simulink model "Adder8bit"  (R2016a)
settings: Solver=VariableStepAuto  StartTime=0.0  StopTime=10.0  RelTol=1e-3
libraries: hdlsllib x17
settings Model: Creator=duyvu  LastModifiedBy=duyvu

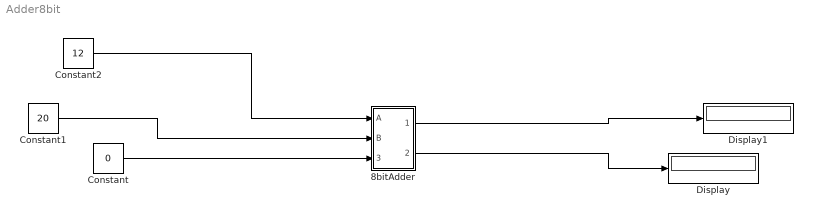
== system Adder8bit ==
  8bitAdder : Subsystem
  Constant : Constant  Value=0  OutDataTypeStr=boolean
  Constant1 : Constant  Value=20  OutDataTypeStr=int8
  Constant2 : Constant  Value=12  OutDataTypeStr=int8
  Display : Display
  Display1 : Display
  wires:
  Constant2/1 -> 8bitAdder/1(A)
  Constant1/1 -> 8bitAdder/2(B)
  Constant/1 -> 8bitAdder/3(CIn)
  8bitAdder/1(Carry) -> Display1/1
  8bitAdder/2(Sum) -> Display/1

== system Adder8bit/8bitAdder ==
  A : Inport  OutDataTypeStr=int8
  B : Inport  Port=2
  CIn : Inport  Port=3
  Bit Concat : hdlsllib/HDL Operations/Bit Concat  numInputs=8
  Data Type Conversion : DataTypeConversion  OutDataTypeStr=int8
  Subsystem10 : Subsystem
  Carry : Outport
  Sum : Outport  Port=2
  wires:
  Data Type Conversion/1 -> Sum/1
  Bit Concat/1 -> Data Type Conversion/1
  Subsystem10/2(Carry) -> Carry/1
  Subsystem10/5(Out3) -> Bit Concat/5
  Subsystem10/6(Out4) -> Bit Concat/4
  Subsystem10/7(Out5) -> Bit Concat/3
  Subsystem10/3(Out1) -> Bit Concat/7
  Subsystem10/4(Out2) -> Bit Concat/6
  B/1 -> Subsystem10/2(B)
  CIn/1 -> Subsystem10/3(CIn)
  A/1 -> Subsystem10/1(A)
  Subsystem10/1(Out0) -> Bit Concat/8
  Subsystem10/8(Out6) -> Bit Concat/2
  Subsystem10/9(Out7) -> Bit Concat/1

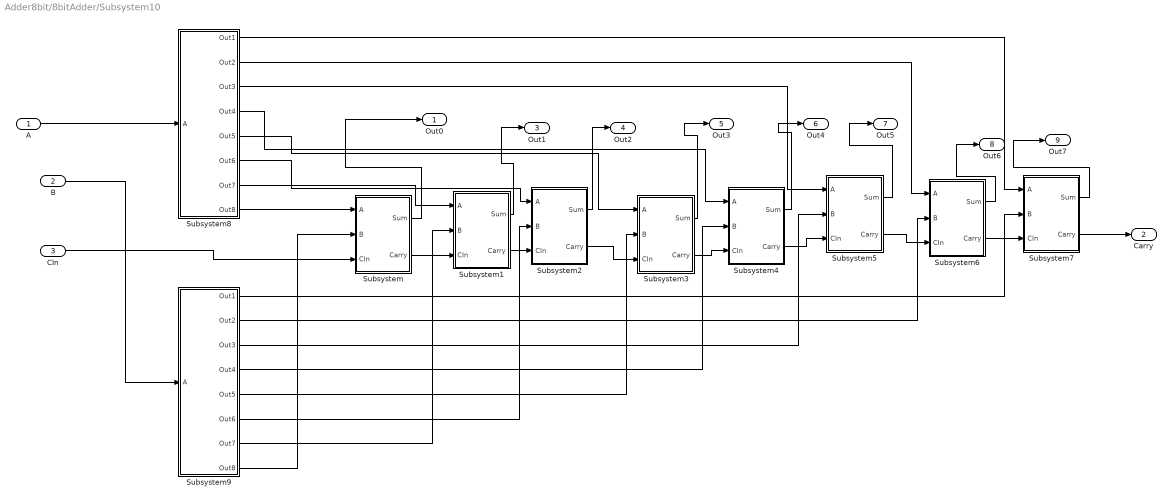
== system Adder8bit/8bitAdder/Subsystem10 ==
  A : Inport  OutDataTypeStr=int8
  B : Inport  Port=2
  CIn : Inport  Port=3
  Subsystem : Subsystem
  Subsystem1 : Subsystem
  Subsystem2 : Subsystem
  Subsystem3 : Subsystem
  Subsystem4 : Subsystem
  Subsystem5 : Subsystem
  Subsystem6 : Subsystem
  Subsystem7 : Subsystem
  Subsystem8 : Subsystem
  Subsystem9 : Subsystem
  Out0 : Outport  OutDataTypeStr=boolean
  Carry : Outport  Port=2
  Out1 : Outport  Port=3  OutDataTypeStr=boolean
  Out2 : Outport  Port=4  OutDataTypeStr=boolean
  Out3 : Outport  Port=5
  Out4 : Outport  Port=6
  Out5 : Outport  Port=7
  Out6 : Outport  Port=8
  Out7 : Outport  Port=9
  wires:
  B/1 -> Subsystem9/1(A)
  Subsystem8/3(Out3) -> Subsystem5/1(A)
  Subsystem8/2(Out2) -> Subsystem6/1(A)
  Subsystem8/7(Out7) -> Subsystem1/1(A)
  Subsystem8/5(Out5) -> Subsystem3/1(A)
  Subsystem8/8(Out8) -> Subsystem/1(A)
  Subsystem8/6(Out6) -> Subsystem2/1(A)
  Subsystem8/4(Out4) -> Subsystem4/1(A)
  Subsystem3/1(Sum) -> Out3/1
  A/1 -> Subsystem8/1(A)
  Subsystem6/1(Sum) -> Out6/1
  Subsystem9/5(Out5) -> Subsystem3/2(B)
  Subsystem5/1(Sum) -> Out5/1
  Subsystem4/1(Sum) -> Out4/1
  Subsystem8/1(Out1) -> Subsystem7/1(A)
  Subsystem7/1(Sum) -> Out7/1
  Subsystem9/8(Out8) -> Subsystem/2(B)
  Subsystem9/4(Out4) -> Subsystem4/2(B)
  Subsystem7/2(Carry) -> Carry/1
  Subsystem/2(Carry) -> Subsystem1/3(CIn)
  Subsystem1/1(Sum) -> Out1/1
  Subsystem2/2(Carry) -> Subsystem3/3(CIn)
  Subsystem1/2(Carry) -> Subsystem2/3(CIn)
  Subsystem/1(Sum) -> Out0/1
  CIn/1 -> Subsystem/3(CIn)
  Subsystem2/1(Sum) -> Out2/1
  Subsystem3/2(Carry) -> Subsystem4/3(CIn)
  Subsystem9/7(Out7) -> Subsystem1/2(B)
  Subsystem9/6(Out6) -> Subsystem2/2(B)
  Subsystem4/2(Carry) -> Subsystem5/3(CIn)
  Subsystem9/1(Out1) -> Subsystem7/2(B)
  Subsystem9/2(Out2) -> Subsystem6/2(B)
  Subsystem9/3(Out3) -> Subsystem5/2(B)
  Subsystem5/2(Carry) -> Subsystem6/3(CIn)
  Subsystem6/2(Carry) -> Subsystem7/3(CIn)

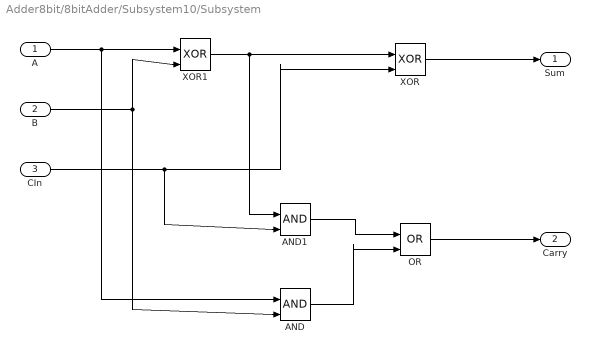
== system Adder8bit/8bitAdder/Subsystem10/Subsystem ==
  A : Inport
  B : Inport  Port=2
  CIn : Inport  Port=3
  AND : Logic  IconShape=distinctive  AllPortsSameDT=off  OutDataTypeStr=boolean
  AND1 : Logic  IconShape=distinctive  AllPortsSameDT=off  OutDataTypeStr=boolean
  "OR " : Logic  Operator=OR  IconShape=distinctive  AllPortsSameDT=off  OutDataTypeStr=boolean
  XOR : Logic  Operator=XOR  IconShape=distinctive  AllPortsSameDT=off  OutDataTypeStr=boolean
  XOR1 : Logic  Operator=XOR  IconShape=distinctive  AllPortsSameDT=off  OutDataTypeStr=boolean
  Sum : Outport
  Carry : Outport  Port=2
  wires:
  CIn/1 -> XOR/2, AND1/2
  XOR1/1 -> AND1/1, XOR/1
  A/1 -> XOR1/1, AND/1
  AND1/1 -> "OR "/1
  XOR/1 -> Sum/1
  B/1 -> AND/2, XOR1/2
  "OR "/1 -> Carry/1
  AND/1 -> "OR "/2

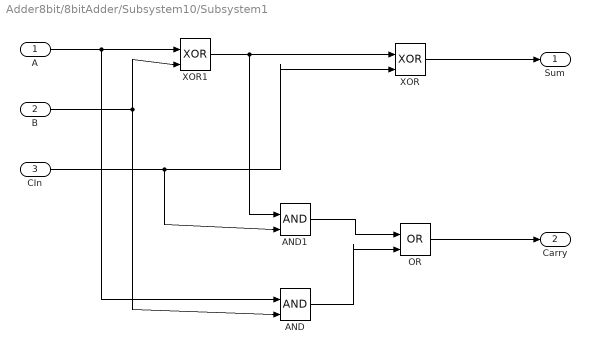
== system Adder8bit/8bitAdder/Subsystem10/Subsystem1 ==
  A : Inport
  B : Inport  Port=2
  CIn : Inport  Port=3
  AND : Logic  IconShape=distinctive  AllPortsSameDT=off  OutDataTypeStr=boolean
  AND1 : Logic  IconShape=distinctive  AllPortsSameDT=off  OutDataTypeStr=boolean
  "OR " : Logic  Operator=OR  IconShape=distinctive  AllPortsSameDT=off  OutDataTypeStr=boolean
  XOR : Logic  Operator=XOR  IconShape=distinctive  AllPortsSameDT=off  OutDataTypeStr=boolean
  XOR1 : Logic  Operator=XOR  IconShape=distinctive  AllPortsSameDT=off  OutDataTypeStr=boolean
  Sum : Outport
  Carry : Outport  Port=2
  wires:
  CIn/1 -> XOR/2, AND1/2
  XOR1/1 -> AND1/1, XOR/1
  A/1 -> XOR1/1, AND/1
  AND1/1 -> "OR "/1
  XOR/1 -> Sum/1
  B/1 -> AND/2, XOR1/2
  "OR "/1 -> Carry/1
  AND/1 -> "OR "/2

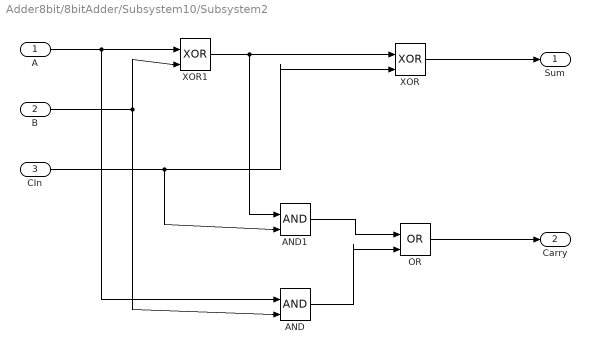
== system Adder8bit/8bitAdder/Subsystem10/Subsystem2 ==
  A : Inport
  B : Inport  Port=2
  CIn : Inport  Port=3
  AND : Logic  IconShape=distinctive  AllPortsSameDT=off  OutDataTypeStr=boolean
  AND1 : Logic  IconShape=distinctive  AllPortsSameDT=off  OutDataTypeStr=boolean
  "OR " : Logic  Operator=OR  IconShape=distinctive  AllPortsSameDT=off  OutDataTypeStr=boolean
  XOR : Logic  Operator=XOR  IconShape=distinctive  AllPortsSameDT=off  OutDataTypeStr=boolean
  XOR1 : Logic  Operator=XOR  IconShape=distinctive  AllPortsSameDT=off  OutDataTypeStr=boolean
  Sum : Outport
  Carry : Outport  Port=2
  wires:
  CIn/1 -> XOR/2, AND1/2
  XOR1/1 -> AND1/1, XOR/1
  A/1 -> XOR1/1, AND/1
  AND1/1 -> "OR "/1
  XOR/1 -> Sum/1
  B/1 -> AND/2, XOR1/2
  "OR "/1 -> Carry/1
  AND/1 -> "OR "/2

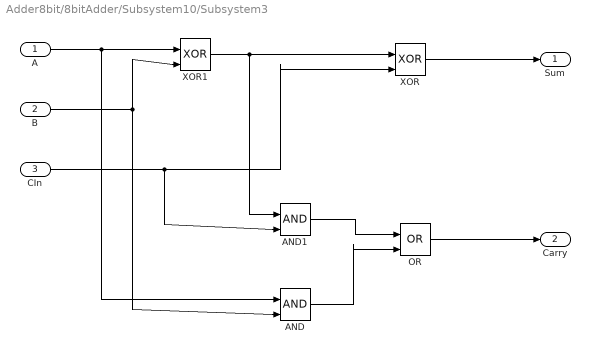
== system Adder8bit/8bitAdder/Subsystem10/Subsystem3 ==
  A : Inport
  B : Inport  Port=2
  CIn : Inport  Port=3
  AND : Logic  IconShape=distinctive  AllPortsSameDT=off  OutDataTypeStr=boolean
  AND1 : Logic  IconShape=distinctive  AllPortsSameDT=off  OutDataTypeStr=boolean
  "OR " : Logic  Operator=OR  IconShape=distinctive  AllPortsSameDT=off  OutDataTypeStr=boolean
  XOR : Logic  Operator=XOR  IconShape=distinctive  AllPortsSameDT=off  OutDataTypeStr=boolean
  XOR1 : Logic  Operator=XOR  IconShape=distinctive  AllPortsSameDT=off  OutDataTypeStr=boolean
  Sum : Outport
  Carry : Outport  Port=2
  wires:
  CIn/1 -> XOR/2, AND1/2
  XOR1/1 -> AND1/1, XOR/1
  A/1 -> XOR1/1, AND/1
  AND1/1 -> "OR "/1
  XOR/1 -> Sum/1
  B/1 -> AND/2, XOR1/2
  "OR "/1 -> Carry/1
  AND/1 -> "OR "/2

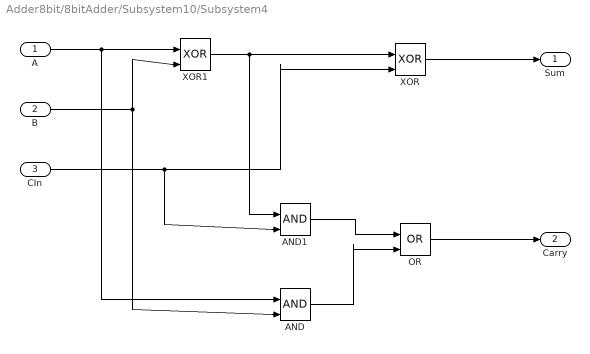
== system Adder8bit/8bitAdder/Subsystem10/Subsystem4 ==
  A : Inport
  B : Inport  Port=2
  CIn : Inport  Port=3
  AND : Logic  IconShape=distinctive  AllPortsSameDT=off  OutDataTypeStr=boolean
  AND1 : Logic  IconShape=distinctive  AllPortsSameDT=off  OutDataTypeStr=boolean
  "OR " : Logic  Operator=OR  IconShape=distinctive  AllPortsSameDT=off  OutDataTypeStr=boolean
  XOR : Logic  Operator=XOR  IconShape=distinctive  AllPortsSameDT=off  OutDataTypeStr=boolean
  XOR1 : Logic  Operator=XOR  IconShape=distinctive  AllPortsSameDT=off  OutDataTypeStr=boolean
  Sum : Outport
  Carry : Outport  Port=2
  wires:
  CIn/1 -> XOR/2, AND1/2
  XOR1/1 -> AND1/1, XOR/1
  A/1 -> XOR1/1, AND/1
  AND1/1 -> "OR "/1
  XOR/1 -> Sum/1
  B/1 -> AND/2, XOR1/2
  "OR "/1 -> Carry/1
  AND/1 -> "OR "/2

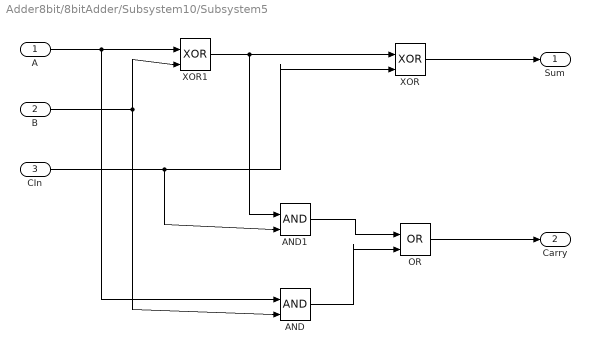
== system Adder8bit/8bitAdder/Subsystem10/Subsystem5 ==
  A : Inport
  B : Inport  Port=2
  CIn : Inport  Port=3
  AND : Logic  IconShape=distinctive  AllPortsSameDT=off  OutDataTypeStr=boolean
  AND1 : Logic  IconShape=distinctive  AllPortsSameDT=off  OutDataTypeStr=boolean
  "OR " : Logic  Operator=OR  IconShape=distinctive  AllPortsSameDT=off  OutDataTypeStr=boolean
  XOR : Logic  Operator=XOR  IconShape=distinctive  AllPortsSameDT=off  OutDataTypeStr=boolean
  XOR1 : Logic  Operator=XOR  IconShape=distinctive  AllPortsSameDT=off  OutDataTypeStr=boolean
  Sum : Outport
  Carry : Outport  Port=2
  wires:
  CIn/1 -> XOR/2, AND1/2
  XOR1/1 -> AND1/1, XOR/1
  A/1 -> XOR1/1, AND/1
  AND1/1 -> "OR "/1
  XOR/1 -> Sum/1
  B/1 -> AND/2, XOR1/2
  "OR "/1 -> Carry/1
  AND/1 -> "OR "/2

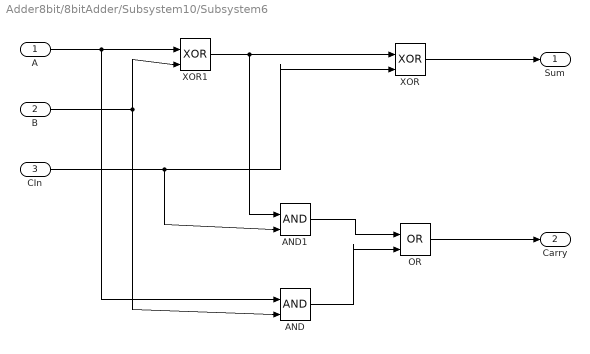
== system Adder8bit/8bitAdder/Subsystem10/Subsystem6 ==
  A : Inport
  B : Inport  Port=2
  CIn : Inport  Port=3
  AND : Logic  IconShape=distinctive  AllPortsSameDT=off  OutDataTypeStr=boolean
  AND1 : Logic  IconShape=distinctive  AllPortsSameDT=off  OutDataTypeStr=boolean
  "OR " : Logic  Operator=OR  IconShape=distinctive  AllPortsSameDT=off  OutDataTypeStr=boolean
  XOR : Logic  Operator=XOR  IconShape=distinctive  AllPortsSameDT=off  OutDataTypeStr=boolean
  XOR1 : Logic  Operator=XOR  IconShape=distinctive  AllPortsSameDT=off  OutDataTypeStr=boolean
  Sum : Outport
  Carry : Outport  Port=2
  wires:
  CIn/1 -> XOR/2, AND1/2
  XOR1/1 -> AND1/1, XOR/1
  A/1 -> XOR1/1, AND/1
  AND1/1 -> "OR "/1
  XOR/1 -> Sum/1
  B/1 -> AND/2, XOR1/2
  "OR "/1 -> Carry/1
  AND/1 -> "OR "/2

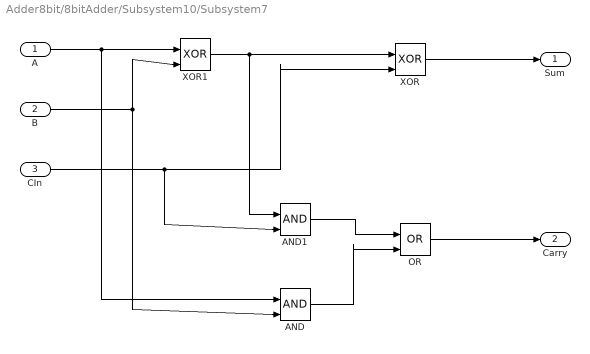
== system Adder8bit/8bitAdder/Subsystem10/Subsystem7 ==
  A : Inport
  B : Inport  Port=2
  CIn : Inport  Port=3
  AND : Logic  IconShape=distinctive  AllPortsSameDT=off  OutDataTypeStr=boolean
  AND1 : Logic  IconShape=distinctive  AllPortsSameDT=off  OutDataTypeStr=boolean
  "OR " : Logic  Operator=OR  IconShape=distinctive  AllPortsSameDT=off  OutDataTypeStr=boolean
  XOR : Logic  Operator=XOR  IconShape=distinctive  AllPortsSameDT=off  OutDataTypeStr=boolean
  XOR1 : Logic  Operator=XOR  IconShape=distinctive  AllPortsSameDT=off  OutDataTypeStr=boolean
  Sum : Outport
  Carry : Outport  Port=2
  wires:
  CIn/1 -> XOR/2, AND1/2
  XOR1/1 -> AND1/1, XOR/1
  A/1 -> XOR1/1, AND/1
  AND1/1 -> "OR "/1
  XOR/1 -> Sum/1
  B/1 -> AND/2, XOR1/2
  "OR "/1 -> Carry/1
  AND/1 -> "OR "/2

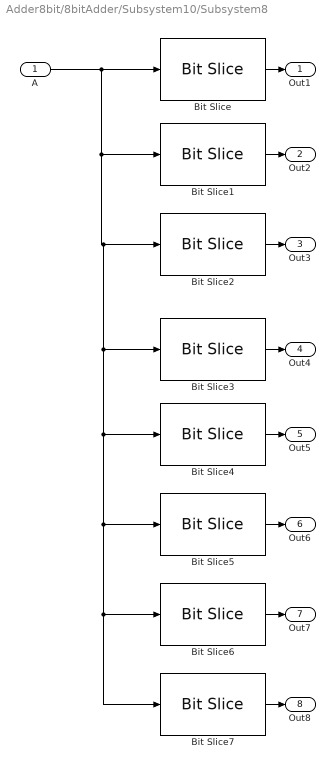
== system Adder8bit/8bitAdder/Subsystem10/Subsystem8 ==
  A : Inport  OutDataTypeStr=int8
  Bit Slice : hdlsllib/HDL Operations/Bit Slice  lidx=7  ridx=7
  Bit Slice1 : hdlsllib/HDL Operations/Bit Slice  lidx=6  ridx=6
  Bit Slice2 : hdlsllib/HDL Operations/Bit Slice  lidx=5  ridx=5
  Bit Slice3 : hdlsllib/HDL Operations/Bit Slice  lidx=4  ridx=4
  Bit Slice4 : hdlsllib/HDL Operations/Bit Slice  lidx=3  ridx=3
  Bit Slice5 : hdlsllib/HDL Operations/Bit Slice  lidx=2  ridx=2
  Bit Slice6 : hdlsllib/HDL Operations/Bit Slice  lidx=1  ridx=1
  Bit Slice7 : hdlsllib/HDL Operations/Bit Slice  lidx=0  ridx=0
  Out1 : Outport
  Out2 : Outport  Port=2
  Out3 : Outport  Port=3
  Out4 : Outport  Port=4
  Out5 : Outport  Port=5
  Out6 : Outport  Port=6
  Out7 : Outport  Port=7
  Out8 : Outport  Port=8
  wires:
  Bit Slice2/1 -> Out3/1
  Bit Slice4/1 -> Out5/1
  Bit Slice/1 -> Out1/1
  Bit Slice1/1 -> Out2/1
  Bit Slice3/1 -> Out4/1
  Bit Slice5/1 -> Out6/1
  Bit Slice6/1 -> Out7/1
  Bit Slice7/1 -> Out8/1
  A/1 -> Bit Slice6/1, Bit Slice7/1, Bit Slice5/1, Bit Slice4/1, Bit Slice3/1, Bit Slice2/1, Bit Slice1/1, Bit Slice/1

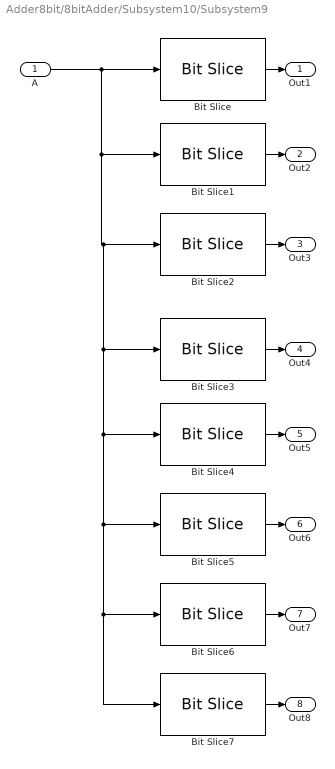
== system Adder8bit/8bitAdder/Subsystem10/Subsystem9 ==
  A : Inport  OutDataTypeStr=int8
  Bit Slice : hdlsllib/HDL Operations/Bit Slice  lidx=7  ridx=7
  Bit Slice1 : hdlsllib/HDL Operations/Bit Slice  lidx=6  ridx=6
  Bit Slice2 : hdlsllib/HDL Operations/Bit Slice  lidx=5  ridx=5
  Bit Slice3 : hdlsllib/HDL Operations/Bit Slice  lidx=4  ridx=4
  Bit Slice4 : hdlsllib/HDL Operations/Bit Slice  lidx=3  ridx=3
  Bit Slice5 : hdlsllib/HDL Operations/Bit Slice  lidx=2  ridx=2
  Bit Slice6 : hdlsllib/HDL Operations/Bit Slice  lidx=1  ridx=1
  Bit Slice7 : hdlsllib/HDL Operations/Bit Slice  lidx=0  ridx=0
  Out1 : Outport
  Out2 : Outport  Port=2
  Out3 : Outport  Port=3
  Out4 : Outport  Port=4
  Out5 : Outport  Port=5
  Out6 : Outport  Port=6
  Out7 : Outport  Port=7
  Out8 : Outport  Port=8
  wires:
  Bit Slice2/1 -> Out3/1
  Bit Slice4/1 -> Out5/1
  Bit Slice/1 -> Out1/1
  Bit Slice1/1 -> Out2/1
  Bit Slice3/1 -> Out4/1
  Bit Slice5/1 -> Out6/1
  Bit Slice6/1 -> Out7/1
  Bit Slice7/1 -> Out8/1
  A/1 -> Bit Slice6/1, Bit Slice7/1, Bit Slice5/1, Bit Slice4/1, Bit Slice3/1, Bit Slice2/1, Bit Slice1/1, Bit Slice/1
